simulink model "TVModel_Simulation_21"  (R2021b)
settings: Solver=FixedStepDiscrete  StartTime=0.0  StopTime=250  FixedStep=0.02  MaxStep=0.01  RelTol=1e-3
undefined symbols (not defined in the file or in its folder): MB, TV, TV_OLD
libraries: simulink x22, simulink_extras x14, eeGeneralControl x13, slpidlib x8, fuzblock x4, controlLib x4, cstblocks x3, dspstat3 x2, eeSlidingModeController x1, sharedTrackingLibrary x1
(part 5 of 9)

== system TVModel_Simulation_21/Subsystem/Subsystem1/Torque Distribution/MPC/ PRE LUDO/Mz = 0 Bound logic ==
  In Bus Element13 : Inport  PortName=brake_signal  Element=regen
  YRD : Inport  Port=2
  In Bus Element1 : Inport  Port=3  PortName=driver_inputs  Element=throttle
  " " : Constant  Value=0.95
  "  " : Constant  Value=TV.LV.GENERAL.ThrottleThresh
  "             " : Constant  Value=TV.LV.GENERAL.YRDTresh
  AND : Logic  IconShape=distinctive  AllPortsSameDT=off  OutDataTypeStr=boolean
  AND1 : Logic  IconShape=distinctive  AllPortsSameDT=off  OutDataTypeStr=boolean
  AND2 : Logic  IconShape=distinctive  AllPortsSameDT=off  OutDataTypeStr=boolean
  Abs : Abs
  Constant : Constant  Value=TV.LV.GENERAL.BrakeThresh
  Constant1 : Constant  Value=10
  Data Type Conversion : DataTypeConversion  OutDataTypeStr=double
  Data Type Conversion1 : DataTypeConversion  OutDataTypeStr=double
  Discrete FIR Filter : DiscreteFir  Coefficients=ones(1,TV.MPC.N/TV.MPC.T*0.2)
  Gain : Gain  Gain=2
  Less Than : RelationalOperator  Operator=<=  OutDataTypeStr=fixdt(1,16)  RndMeth=Simplest
  Less Than1 : RelationalOperator  OutDataTypeStr=boolean  RndMeth=Simplest
  Less Than2 : RelationalOperator  Operator=<  OutDataTypeStr=boolean  RndMeth=Simplest
  Less Than3 : RelationalOperator  Operator=<  OutDataTypeStr=boolean  RndMeth=Simplest
  Less Than4 : RelationalOperator  OutDataTypeStr=boolean  RndMeth=Simplest
  Sum : Sum
  flag : Outport
  wires:
  Less Than/1 -> Discrete FIR Filter/1
  Constant1/1 -> Less Than4/2
  Less Than4/1 -> AND/1, AND1/2
  Discrete FIR Filter/1 -> Less Than4/1
  "  "/1 -> Less Than1/2
  "             "/1 -> Less Than/2
  Abs/1 -> Less Than/1
  YRD/1 -> Abs/1
  In Bus Element1/1 -> Less Than1/1
  Less Than1/1 -> AND/2
  In Bus Element13/1 -> Less Than3/2, Less Than2/1
  " "/1 -> Less Than2/2
  AND1/1 -> Data Type Conversion1/1
  Gain/1 -> Sum/1
  AND/1 -> Data Type Conversion/1
  Sum/1 -> flag/1
  Data Type Conversion/1 -> Sum/2
  Data Type Conversion1/1 -> Gain/1
  AND2/1 -> AND1/1
  Less Than2/1 -> AND2/1
  Less Than3/1 -> AND2/2
  Constant/1 -> Less Than3/1

== system TVModel_Simulation_21/Subsystem/Subsystem1/Torque Distribution/MPC/ PRE LUDO/Power Calculation Post ==
  Motor_Torque : Inport  OutDataTypeStr=double  PortDimensions=4
  In Bus Element34 : Inport  Port=2  PortName=dynamics_data  Element=omega_wheels
  In Bus Element2 : Inport  Port=2  PortName=dynamics_data  Element=omega_wheels
  "     " : Gain  Gain=TV.LV.inv_efficiency
  "      " : Gain  Gain=1/TV.LV.inv_efficiency
  Divide : Product  Inputs=*/*
  Gain2 : Gain  Gain=TV.CAR.Tau
  Power to engines : Subsystem
  Saturation : Saturate  UpperLimit=19900*pi/30  LowerLimit=100*pi/30
  Sum of Elements : Sum  Inputs=+
  Switch3 : Switch  Criteria=u2 > Threshold
  Terminator : Terminator
  wires:
  Divide/1 -> Sum of Elements/1
  Saturation/1 -> Divide/1, Power to engines/1(omega_motor)
  Power to engines/1(Efficiency) -> "      "/1, "     "/1
  "      "/1 -> Switch3/3  "Braking"
  "     "/1 -> Switch3/1  "Driving"
  Motor_Torque/1 -> Power to engines/2(Torque), Divide/3
  In Bus Element34/1 -> Gain2/1
  Gain2/1 -> Saturation/1
  In Bus Element2/1 -> Switch3/2
  Switch3/1 -> Divide/2
  Sum of Elements/1 -> Terminator/1  "p_el_post"

== system TVModel_Simulation_21/Subsystem/Subsystem1/Torque Distribution/MPC/ PRE LUDO/Power Calculation Pre ==
  Motor_Torque : Inport  OutDataTypeStr=double  PortDimensions=4
  In Bus Element34 : Inport  Port=2  PortName=dynamics_data  Element=omega_wheels
  In Bus Element2 : Inport  Port=2  PortName=dynamics_data  Element=omega_wheels
  "     " : Gain  Gain=TV.LV.inv_efficiency
  "      " : Gain  Gain=1/TV.LV.inv_efficiency
  Divide : Product  Inputs=*/*
  Gain2 : Gain  Gain=TV.CAR.Tau
  Power to engines : Subsystem
  Saturation : Saturate  UpperLimit=19900*pi/30  LowerLimit=100*pi/30
  Sum of Elements : Sum  Inputs=+
  Switch3 : Switch  Criteria=u2 > Threshold
  Terminator : Terminator
  wires:
  Power to engines/1(Efficiency) -> "      "/1, "     "/1
  "      "/1 -> Switch3/3  "Braking"
  "     "/1 -> Switch3/1  "Driving"
  Motor_Torque/1 -> Divide/3, Power to engines/2(Torque)
  In Bus Element34/1 -> Gain2/1
  Gain2/1 -> Saturation/1
  In Bus Element2/1 -> Switch3/2
  Sum of Elements/1 -> Terminator/1  "p_el_pre"
  Saturation/1 -> Divide/1, Power to engines/1(omega_motor)
  Switch3/1 -> Divide/2
  Divide/1 -> Sum of Elements/1

== system TVModel_Simulation_21/Subsystem/Subsystem1/Torque Distribution/MPC/ PRE LUDO/Steer_activation ==
  front_wheel_angle : Inport
  Constant : Constant  Value=TV.SIGNALS.SETTINGS.MzLimit
  Product : Product
  Steer Activation : Subsystem
  Mz_Lim : Outport
  wires:
  Constant/1 -> Product/2
  Steer Activation/1(epsilon) -> Product/1  "epsilon"
  Product/1 -> Mz_Lim/1  "Mz_Lim"
  front_wheel_angle/1 -> Steer Activation/1(front_wheel_angle)

== system TVModel_Simulation_21/Subsystem/Subsystem1/Torque Distribution/MPC/ Parameter Bus /Bus p ==
  In : Inport
  C Function : CFunction  OutputCode=|
      | int i,j;
      | for (i = 0; i < N; i++) {
      |  for (j = 0; j < np; j++) {
      |   out_x[i*np+j] = in_x[j];
      |  }
      | }
  Constant1 : Constant  Value=TV.MPC.N + 1  OutDataTypeStr=uint8  SampleTime=TV.MPC.T/TV.MPC.N
  Constant3 : Constant  Value=TV.MPC.np  OutDataTypeStr=uint8  SampleTime=TV.MPC.T/TV.MPC.N
  Rate Transition3 : RateTransition  OutPortSampleTime=TV.MPC.T/TV.MPC.N
  TV_Info : Outport
  wires:
  Constant1/1 -> C Function/2
  C Function/1 -> TV_Info/1
  Constant3/1 -> C Function/3
  Rate Transition3/1 -> C Function/1
  In/1 -> Rate Transition3/1

== system TVModel_Simulation_21/Subsystem/Subsystem1/Torque Distribution/MPC/Faults Detection/MPC ==
  X1 : Inport
  Action Port : ActionPort  ActionPortLabel=if(u1 == 1)
  Out1 : Outport
  wires:
  X1/1 -> Out1/1

== system TVModel_Simulation_21/Subsystem/Subsystem1/Torque Distribution/MPC/Faults Detection/Simple torque ==
  In Bus Element11 : Inport  PortName=driver_inputs
  In Bus Element10 : Inport  Port=2  PortName=dynamics_data
  In Bus Element13 : Inport  Port=3  PortName=brake_signal
  In Bus Element12 : Inport  Port=4  PortName=hv
  In Bus torque_map1 : Inport  Port=5  PortName=car_settings
  Bus Element In : Inport  Port=6  PortName=Tire_Bounds
  Action Port : ActionPort  ActionPortLabel=elseif(u1 == 2)
  No_TV : Subsystem
  Out1 : Outport
  wires:
  Bus Element In/1 -> No_TV/6(Tire_Bounds)
  No_TV/1(Output) -> Out1/1
  In Bus Element11/1 -> No_TV/4(driver_inputs)
  In Bus Element10/1 -> No_TV/1(dynamics_data)
  In Bus Element12/1 -> No_TV/3(hv)
  In Bus Element13/1 -> No_TV/2(brake_signal)
  In Bus torque_map1/1 -> No_TV/5(car_settings)

== system TVModel_Simulation_21/Subsystem/Subsystem1/Torque Distribution/MPC/Faults Detection/Subsystem ==
  OCP Status : Inport
  In Bus Element2 : Inport  Port=2  PortName=dynamics_data  Element=vx
  Backup Map : Subsystem  TreatAsAtomicUnit=on
  Constant : Constant  Value=2
  Constant1 : Constant  Value=TV.MPC.N/TV.MPC.T*0.1-1
  Constant2 : Constant  Value=4
  Data Type Conversion : DataTypeConversion  OutDataTypeStr=uint8  RndMeth=Nearest
  Discrete FIR Filter : DiscreteFir  Coefficients=ones(1,TV.MPC.N/TV.MPC.T*0.1)
  Equal : RelationalOperator  Operator===  OutDataTypeStr=boolean  RndMeth=Simplest
  If : If  IfExpression=u1 == 0
  Less Than1 : RelationalOperator  OutDataTypeStr=boolean  RndMeth=Simplest
  Merge : Merge
  Selected Map : Subsystem  TreatAsAtomicUnit=on
  Switch : Switch  Criteria=u2 > Threshold  Threshold=TV.LV.GENERAL.VxTresh
  TV Mode Selection : Outport
  wires:
  Data Type Conversion/1 -> Discrete FIR Filter/1
  Constant2/1 -> Equal/2
  OCP Status/1 -> Equal/1
  Equal/1 -> Data Type Conversion/1
  Constant/1 -> Switch/3
  Switch/1 -> TV Mode Selection/1
  In Bus Element2/1 -> Switch/2
  Merge/1 -> Switch/1
  Discrete FIR Filter/1 -> Less Than1/1
  Constant1/1 -> Less Than1/2
  Less Than1/1 -> If/1
  If/1 -> Selected Map/Action
  Selected Map/1(Out1) -> Merge/1
  If/2 -> Backup Map/Action
  Backup Map/1(Out1) -> Merge/2

== system TVModel_Simulation_21/Subsystem/Subsystem1/Torque Distribution/MPC/Mz Generation/Steer Activation ==
  front_wheel_angle : Inport
  In Bus Element2 : Inport  Port=2  PortName=dynamics_data  Element=vx
  AND : Logic  Commented=on  IconShape=distinctive  AllPortsSameDT=off  OutDataTypeStr=boolean
  AND1 : Logic  Commented=on  IconShape=distinctive  AllPortsSameDT=off  OutDataTypeStr=boolean
  Abs : Abs
  Constant : Constant  Commented=on  Value=TV.LV.GENERAL.VxTresh
  Constant1 : Constant  Value=2*pi/180
  Constant4 : Constant  Value=pi/180/2
  Delay : Delay  Commented=on  DelayLength=5
  First Activation : Subsystem  Commented=on
  If : If  Commented=on  IfExpression=u1 == 1
  If Action Subsystem : Subsystem  Commented=on  TreatAsAtomicUnit=on
  If Action Subsystem1 : Subsystem  Commented=on  TreatAsAtomicUnit=on
  Less Than : RelationalOperator  Operator=<=  OutDataTypeStr=boolean  RndMeth=Simplest
  Less Than1 : RelationalOperator  Commented=on  OutDataTypeStr=boolean  RndMeth=Simplest
  Less Than2 : RelationalOperator  Operator=<  OutDataTypeStr=boolean  RndMeth=Simplest
  Merge : Merge  Commented=on
  S-R Flip-Flop : simulink_extras/Flip Flops/S-R Flip-Flop  initial_condition=0
  Terminator : Terminator
  epsilon : Outport
  wires:
  If/1 -> If Action Subsystem1/Action
  If Action Subsystem/1(Epsilon) -> Merge/2
  If Action Subsystem1/1(epsilon) -> Merge/1
  First Activation/1(OUt) -> If/1  "u1"
  S-R Flip-Flop/1 -> First Activation/1(In), epsilon/1, If Action Subsystem1/1(Inport), Delay/1, If Action Subsystem/1(Inport)  "Q"
  If/2 -> If Action Subsystem/Action
  front_wheel_angle/1 -> Abs/1
  Constant1/1 -> Less Than/1
  S-R Flip-Flop/2 -> Terminator/1
  Less Than2/1 -> S-R Flip-Flop/2, AND/1  "reset"
  Less Than/1 -> S-R Flip-Flop/1  "set"
  Delay/1 -> AND/2
  Abs/1 -> Less Than/2, Less Than2/1
  Constant4/1 -> Less Than2/2
  Merge/1 -> AND1/1  "epsilon"
  Less Than1/1 -> AND1/2
  Constant/1 -> Less Than1/2
  In Bus Element2/1 -> Less Than1/1

== system TVModel_Simulation_21/Subsystem/Subsystem1/Torque Distribution/MPC/Polytopic Constraints/Driver Inputs ==
  In Bus Element35 : Inport  PortName=brake_signal  Element=regen
  In Bus Element2 : Inport  Port=2  PortName=driver_inputs  Element=throttle
  In Bus torque_map : Inport  Port=3  PortName=Car_Settings  Element=torque_map
  Bus Element In1 : Inport  Port=4  PortName=ubx  Element=ubx
  Bus Element In2 : Inport  Port=4  PortName=ubx  Element=lbx
  " " : Logic  Operator=XOR  IconShape=distinctive  AllPortsSameDT=off  OutDataTypeStr=boolean
  "Accelerator Mapping " : Subsystem
      settings: PortSchema="{\"entries\":[{\"content\":{\"sides\":[{\"content\":{\"connectorIds\":[\"In1\"]},\"type\":\"ConnectorPlacement.EquallySpacedRectSide\",\"uuid\":\"12eec289-8173-4d00-9637-a8f11e8894d3\"},{\"content\":{\"connectorIds\":[\"Out1\"],\"side\":\"RIGHT\"},\"type\":\"ConnectorPlacement.EquallySpacedRectSide\",\"uuid\":\"db75e905-0694-4773-89a3-439123e45b7e\"},{\"content\":{\"connectorIds\":[\"Out2\"],\"side\":\"TOP\"},\"type\":\"ConnectorPlacement.EquallySpacedRectSide\",\"uuid\":\"1c38e3d9-f7d7-40f1-94e6-0479f4c62d9d\"}]},\"type\":\"ConnectorPlacement.EquallySpacedConnector\",\"uuid\":\"6d4996fb-8621-4156-91e1-8a66b5180382\"}],\"packageUris\":[\"http://schema.mathworks.com/mf0/Connector/R2020b\"],\"version\":\"1.0\"}"
  Constant1 : Constant  Value=TV.LV.GENERAL.BrakeThresh
  Constant10 : Constant  Value=TV.LV.TORQUE.T_nominal_motor
  Constant2 : Constant  Value=TV.LV.GENERAL.ThrottleThresh
  Constant9 : Constant  Value=TV.LV.TORQUE.T_peak_motor
  Gain1 : Gain  Gain=4
  Gain2 : Gain  Gain=0.99
  Gain3 : Gain
  Less Than : RelationalOperator  OutDataTypeStr=boolean  RndMeth=Simplest
  Less Than1 : RelationalOperator  OutDataTypeStr=boolean  RndMeth=Simplest
  MATLAB Function3 : MATLAB Function  TreatAsAtomicUnit=on
  MATLAB Function4 : MATLAB Function  TreatAsAtomicUnit=on
  Multiport Switch1 : MultiPortSwitch  DataPortOrder=Specify indices  Inputs={TV.LV.TORQUE.T_peak_setting,TV.LV.TORQUE.T_nominal_setting}  DataPortIndices={TV.LV.TORQUE.T_peak_setting,TV.LV.TORQUE.T_nominal_setting}
  Product : Product
  Product1 : Product
  Saturation Dynamic : simulink/Discontinuities/Saturation Dynamic  OutMin=[]  OutMax=[]  OutDataTypeStr=Inherit: Same as second input  OutDataType=fixdt(1, 16)  OutScaling=2^-10  DoSatur=off
  Subtract1 : Sum  Inputs=+-
  Out Bus Element : Outport  PortName=percentage  Element=95
  Out Bus Element1 : Outport  PortName=percentage  Element=105
  Out Bus Element2 : Outport  Port=2  PortName=TV_Info  Element=Accelerator_Mapping
  wires:
  Product1/1 -> Product/1
  " "/1 -> Product1/1
  Constant9/1 -> Multiport Switch1/2
  Product/1 -> Saturation Dynamic/2  "g_requested"
  Subtract1/1 -> Product1/2
  Multiport Switch1/1 -> Gain1/1
  Constant10/1 -> Multiport Switch1/3
  Constant2/1 -> Less Than1/2
  "Accelerator Mapping "/1(mapped_acc) -> Subtract1/1
  In Bus torque_map/1 -> Multiport Switch1/1
  In Bus Element35/1 -> Less Than/1, Subtract1/2  "regen"
  Less Than1/1 -> " "/2
  Constant1/1 -> Less Than/2
  In Bus Element2/1 -> "Accelerator Mapping "/1(acc), Less Than1/1
  Less Than/1 -> " "/1
  Gain1/1 -> Product/2
  "Accelerator Mapping "/2(TV_Info) -> Out Bus Element2/1
  Gain3/1 -> Out Bus Element1/1
  MATLAB Function4/1(ug_saturation) -> Saturation Dynamic/1
  Bus Element In2/1 -> MATLAB Function3/1(lbx)
  MATLAB Function3/1(lg_saturation) -> Saturation Dynamic/3
  Saturation Dynamic/1 -> Gain3/1, Gain2/1  "yg"
  Gain2/1 -> Out Bus Element/1
  Bus Element In1/1 -> MATLAB Function4/1(ubx)

== system TVModel_Simulation_21/Subsystem/Subsystem1/Torque Distribution/MPC/Polytopic Constraints/Driver g ==
  In Bus Element1 : Inport  PortName=brake_signal
  In Bus Element : Inport  Port=2  PortName=percentage  Element=95
  In Bus Element2 : Inport  Port=2  PortName=percentage  Element=95
  In Bus Element4 : Inport  Port=2  PortName=percentage  Element=105
  In Bus Element5 : Inport  Port=2  PortName=percentage  Element=105
  In Bus Element3 : Inport  Port=3  PortName=driver_inputs
  Coasting : Subsystem
      settings: PortSchema="{\"entries\":[{\"content\":{\"sides\":[{\"content\":{\"connectorIds\":[\"In1\",\"In2\"]},\"type\":\"ConnectorPlacement.EquallySpacedRectSide\",\"uuid\":\"12822615-03ad-45f6-8c43-45acae00b3c9\"},{\"content\":{\"connectorIds\":[\"Out1\"],\"side\":\"RIGHT\"},\"type\":\"ConnectorPlacement.EquallySpacedRectSide\",\"uuid\":\"651d1d31-9a4c-422b-aacb-e7edf3ade298\"},{\"content\":{\"connectorIds\":[\"Out2\"],\"side\":\"TOP\"},\"type\":\"ConnectorPlacement.EquallySpacedRectSide\",\"uuid\":\"d0f71465-89ce-4a1f-947c-d935b63c1581\"}]},\"type\":\"ConnectorPlacement.EquallySpacedConnector\",\"uuid\":\"d07c68d3-c928-4ca4-a746-c386ba32e252\"}],\"packageUris\":[\"http://schema.mathworks.com/mf0/Connector/R2020b\"],\"version\":\"1.0\"}"
  Engine Brake : Constant  Value=-TV.SIGNALS.SETTINGS.EngineBrake*TV.LV.TORQUE.T_nominal_motor*4
  Max : MinMax  Function=max  Inputs=2
  Max1 : MinMax  Inputs=2
  Switch2 : Switch  Criteria=u2 > Threshold
  ug_driver : Outport
  lg_driver : Outport  Port=2
  Out Bus Element1 : Outport  Port=3  PortName=TV_Info  Element=Coasting
  wires:
  In Bus Element3/1 -> Coasting/1(driver_inputs)
  In Bus Element1/1 -> Coasting/2(brake_signal)
  Switch2/1 -> lg_driver/1
  In Bus Element/1 -> Max1/1
  Max1/1 -> Switch2/3
  Engine Brake/1 -> Switch2/1
  Coasting/1(coasting_flag) -> Switch2/2
  In Bus Element2/1 -> Max/1
  In Bus Element4/1 -> Max1/2
  In Bus Element5/1 -> Max/2
  Coasting/2(TV_Info) -> Out Bus Element1/1
  Max/1 -> ug_driver/1

== system TVModel_Simulation_21/Subsystem/Subsystem1/Torque Distribution/MPC/Polytopic Constraints/Power Limits Negative ==
  In Bus Element5 : Inport  PortName=hv  Element=cooling.battery.Power_limits [W]
  Gain : Gain  Gain=1/1000
  IC : InitialCondition  Value=-35000
  Max Regen : Saturate  UpperLimit=40000  LowerLimit=0
  Selector : Selector  InputPortWidth=2  IndexOptions=Index vector (dialog)  Indices=[1]  OutputSizes=1
  Unary Minus1 : UnaryMinus
  lg_power : Outport
  wires:
  Unary Minus1/1 -> IC/1  "lPowerLimit"
  Max Regen/1 -> Unary Minus1/1
  In Bus Element5/1 -> Selector/1
  Selector/1 -> Max Regen/1
  IC/1 -> Gain/1
  Gain/1 -> lg_power/1

== system TVModel_Simulation_21/Subsystem/Subsystem1/Torque Distribution/MPC/Polytopic Constraints/Power Limits Positive ==
  In Bus Element5 : Inport  PortName=hv  Element=cooling.battery.Power_limits [W]
  Gain : Gain  Gain=1/1000
  IC1 : InitialCondition  Value=80000
  Selector1 : Selector  InputPortWidth=2  IndexOptions=Index vector (dialog)  Indices=[2]  OutputSizes=1
  ug_power : Outport
  wires:
  In Bus Element5/1 -> Selector1/1
  Selector1/1 -> IC1/1  "uPowerLimit"
  IC1/1 -> Gain/1
  Gain/1 -> ug_power/1

== system TVModel_Simulation_21/Subsystem/Subsystem1/Torque Distribution/MPC/Polytopic Constraints/Subsystem ==
  Torque : Inport
  Abs1 : Abs
  Abs3 : Abs
  Selector : Selector  InputPortWidth=4  IndexOptions=Index vector (dialog)  Indices=[2]  OutputSizes=1
  Selector1 : Selector  InputPortWidth=4  IndexOptions=Index vector (dialog)  Indices=[1]  OutputSizes=1
  Torque1 : InportShadow
  Right : Outport
  Left : Outport  Port=2
  wires:
  Torque1/1 -> Selector1/1
  Selector1/1 -> Abs3/1
  Selector/1 -> Abs1/1
  Torque/1 -> Selector/1
  Abs1/1 -> Right/1
  Abs3/1 -> Left/1

== system TVModel_Simulation_21/Subsystem/Subsystem1/Torque Distribution/MPC/Polytopic Constraints/Subsystem1 ==
  Torque : Inport
  Abs1 : Abs
  Abs3 : Abs
  Selector : Selector  InputPortWidth=4  IndexOptions=Index vector (dialog)  Indices=[2]  OutputSizes=1
  Selector1 : Selector  InputPortWidth=4  IndexOptions=Index vector (dialog)  Indices=[1]  OutputSizes=1
  Torque1 : InportShadow
  Unary Minus : UnaryMinus
  Unary Minus1 : UnaryMinus
  Right : Outport
  Left : Outport  Port=2
  wires:
  Abs1/1 -> Unary Minus/1
  Torque/1 -> Selector/1
  Selector/1 -> Abs1/1
  Selector1/1 -> Abs3/1
  Torque1/1 -> Selector1/1
  Abs3/1 -> Unary Minus1/1
  Unary Minus/1 -> Right/1
  Unary Minus1/1 -> Left/1

== system TVModel_Simulation_21/Subsystem/Subsystem1/Torque Distribution/MPC/States Constraints/Anti reverse wheelspin ==
  lbx_in : Inport  PortDimensions=4
  In Bus Element4 : Inport  Port=2  PortName=slip_ratio
  In Bus Element1 : Inport  Port=2  PortName=slip_ratio
  Constant : Constant  Value=-0.6
  Constant1 : Constant  Value=-0.3
  Less Than : RelationalOperator  Operator=<=  OutDataTypeStr=boolean  RndMeth=Simplest
  Less Than1 : RelationalOperator  OutDataTypeStr=boolean  RndMeth=Simplest
  NOT : Logic  Operator=NOT  IconShape=distinctive  AllPortsSameDT=off  OutDataTypeStr=boolean
  Product : Product
  S-R Flip Flops : Subsystem
  Terminator : Terminator
  lbx_out : Outport  PortDimensions=4
  wires:
  NOT/1 -> Terminator/1  "AntiWheelSpin_Activation_Flag"
  S-R Flip Flops/1(Out1) -> Product/2, NOT/1
  Less Than1/1 -> S-R Flip Flops/2(Reset)
  Less Than/1 -> S-R Flip Flops/1(Set)
  Constant1/1 -> Less Than1/2
  In Bus Element1/1 -> Less Than1/1
  Product/1 -> lbx_out/1
  lbx_in/1 -> Product/1
  In Bus Element4/1 -> Less Than/1
  Constant/1 -> Less Than/2

== system TVModel_Simulation_21/Subsystem/Subsystem1/Torque Distribution/MPC/States Constraints/Brake & ESP ==
  ubx_in : Inport
  In Bus Element13 : Inport  Port=2  PortName=brake_signal  Element=regen
  Constant : Constant
  Constant1 : Constant  Value=0
  Product : Product
  Switch : Switch  Criteria=u2 > Threshold  Threshold=0.95
  ubx_out : Outport
  wires:
  Product/1 -> ubx_out/1
  Switch/1 -> Product/2
  ubx_in/1 -> Product/1
  Constant1/1 -> Switch/1
  Constant/1 -> Switch/3
  In Bus Element13/1 -> Switch/2

== system TVModel_Simulation_21/Subsystem/Subsystem1/Torque Distribution/MPC/States Constraints/Low YRD ==
  ubx_in : Inport
  lbx_max : Inport  Port=2
  lbx_in : Inport  Port=3
  Demux : Demux
  Demux1 : Demux
  Mux : Mux  Inputs=9
  bounds : Outport
  wires:
  lbx_max/1 -> Mux/5
  Demux/4 -> Mux/4
  Demux/3 -> Mux/3
  Demux/2 -> Mux/2
  Demux/1 -> Mux/1
  ubx_in/1 -> Demux/1
  Mux/1 -> bounds/1
  Demux1/3 -> Mux/8
  lbx_in/1 -> Demux1/1
  Demux1/2 -> Mux/7
  Demux1/4 -> Mux/9
  Demux1/1 -> Mux/6

== system TVModel_Simulation_21/Subsystem/Subsystem1/Torque Distribution/MPC/States Constraints/Tire Bounds ==
  In Bus Element : Inport  PortName=fz
  In Bus Element2 : Inport  PortName=fz
  In Bus Element1 : Inport  Port=2  PortName=slip_angle
  In Bus Element3 : Inport  Port=2  PortName=slip_angle
  In Bus Element4 : Inport  Port=3  PortName=dynamics_data
  2-D Lookup Table : Lookup_n-D  BreakpointsForDimension1=TV.LUT.MPC_Lut.control_bound_dry.Fz  BreakpointsForDimension2=TV.LUT.MPC_Lut.control_bound_dry.alpha  Table=TV.LUT.MPC_Lut.control_bound_dry.Fx_target_positive  InternalRulePriority=Speed  RndMeth=Simplest  InputSameDT=on
      settings: InputPortMap=u0,u1
  2-D Lookup Table1 : Lookup_n-D  BreakpointsForDimension1=TV.LUT.MPC_Lut.control_bound_dry.Fz  BreakpointsForDimension2=TV.LUT.MPC_Lut.control_bound_dry.alpha  Table=TV.LUT.MPC_Lut.control_bound_dry.Fx_target_negative  InternalRulePriority=Speed  RndMeth=Simplest  InputSameDT=on
      settings: InputPortMap=u0,u1
  Gain : Gain  Gain=TV.CAR.rs/TV.CAR.Tau
  Gain1 : Gain  Gain=TV.CAR.rs/TV.CAR.Tau
  Hydraulic brakes : Subsystem
  LMUx Correction : Subsystem
      settings: PortSchema="{\"entries\":[{\"content\":{\"sides\":[{\"content\":{\"connectorIds\":[]},\"type\":\"ConnectorPlacement.EquallySpacedRectSide\",\"uuid\":\"3584feb2-5a88-411e-904a-cebd49175db1\"},{\"content\":{\"connectorIds\":[\"Out1\"],\"side\":\"RIGHT\"},\"type\":\"ConnectorPlacement.EquallySpacedRectSide\",\"uuid\":\"3ab4f304-c705-48db-a675-7c67b0246c6a\"},{\"content\":{\"connectorIds\":[\"Out2\"],\"side\":\"TOP\"},\"type\":\"ConnectorPlacement.EquallySpacedRectSide\",\"uuid\":\"35f1ab2e-6666-4377-9bcf-c0062baa00ab\"}]},\"type\":\"ConnectorPlacement.EquallySpacedConnector\",\"uuid\":\"03f15aa2-f62f-4666-8bb4-1f7a61fcffbb\"}],\"packageUris\":[\"http://schema.mathworks.com/mf0/Connector/R2020b\"],\"version\":\"1.0\"}"
  Product : Product
  Product1 : Product
  Saturation : Saturate  UpperLimit=0  LowerLimit=-inf
  Saturation1 : Saturate  UpperLimit=+inf  LowerLimit=0
  tire_ubx : Outport
  tire_lbx : Outport  Port=2
  Out Bus Element1 : Outport  Port=3  PortName=TV_Info  Element=tire_lbx
  Out Bus Element2 : Outport  Port=3  PortName=TV_Info  Element=tire_ubx
  Out Bus Element3 : Outport  Port=3  PortName=TV_Info  Element=LMUx_Correction
  wires:
  In Bus Element/1 -> 2-D Lookup Table/1
  In Bus Element1/1 -> 2-D Lookup Table/2
  In Bus Element2/1 -> 2-D Lookup Table1/1
  In Bus Element3/1 -> 2-D Lookup Table1/2
  Saturation1/1 -> tire_ubx/1, Out Bus Element2/1
  2-D Lookup Table1/1 -> Gain1/1
  In Bus Element4/1 -> Hydraulic brakes/2(dynamics_data)
  Gain1/1 -> Product1/2
  Product/1 -> Saturation1/1
  Gain/1 -> Product/1
  Hydraulic brakes/1(tire_lbx_out) -> Saturation/1
  Product1/1 -> Hydraulic brakes/1(tire_lbx_in)
  LMUx Correction/1(lmux) -> Product/2, Product1/1
  2-D Lookup Table/1 -> Gain/1
  Saturation/1 -> tire_lbx/1, Out Bus Element1/1
  LMUx Correction/2(TV_Info) -> Out Bus Element3/1

== system TVModel_Simulation_21/Subsystem/Subsystem1/Torque Distribution/MPC/USEFUL STUFFFF/Extended Kalman Filter ==
  Motor_Torque : Inport
  In Bus Element4 : Inport  Port=2  PortName=slip_ratio
  In Bus Element : Inport  Port=3  PortName=dynamics_data  Element=vx
  In Bus Element1 : Inport  Port=3  PortName=dynamics_data  Element=vy
  In Bus Element2 : Inport  Port=3  PortName=dynamics_data  Element=yaw_rate
  In Bus Element11 : Inport  Port=4  PortName=front_wheel_angles
  " Parameter Bus " : Subsystem
  Band-Limited White Noise : simulink/Sources/Band-Limited White Noise  Cov=0.00005  Ts=0.01  seed=[23341]
  Band-Limited White Noise1 : simulink/Sources/Band-Limited White Noise  Cov=0.000001  Ts=0.01  seed=[23341]
  Band-Limited White Noise2 : simulink/Sources/Band-Limited White Noise  Cov=0.00001  Ts=0.01  seed=[85]
  Extended Kalman Filter : sharedTrackingLibrary/Extended Kalman Filter  StateTransitionFcn=state_update_kalman  HasStateTransitionJacobianFcn=off  HasAdditiveProcessNoise=Additive  ProcessNoise=diag(0.1*[0.1,0.1,0.1])  HasTimeVaryingProcessNoise=off  HasStateTransitionFcnExtraArgument=1  InitialState=[0,0,0];  InitialStateCovariance=diag(0.1*[0.1,0.1,0.1])  MeasurementFcn1=measurement_kalman  HasMeasurementJacobianFcn1=off  HasMeasurementEnablePort1=off  HasAdditiveMeasurementNoise1=Additive  MeasurementNoise1=diag(0.1*[0.01,0.01,1])  HasTimeVaryingMeasurementNoise1=off  HasMeasurementFcnExtraArgument1=0  HasMeasurementWrapping1=off  MeasurementFcn2=myMeasurementFcn  HasMeasurementJacobianFcn2=off  HasMeasurementEnablePort2=off  HasAdditiveMeasurementNoise2=Additive  MeasurementNoise2=1  HasTimeVaryingMeasurementNoise2=off  HasMeasurementFcnExtraArgument2=0  HasMeasurementWrapping2=off  MeasurementFcn3=myMeasurementFcn  HasMeasurementJacobianFcn3=off  HasMeasurementEnablePort3=off  HasAdditiveMeasurementNoise3=Additive  MeasurementNoise3=1  HasTimeVaryingMeasurementNoise3=off  HasMeasurementFcnExtraArgument3=0  HasMeasurementWrapping3=off  MeasurementFcn4=myMeasurementFcn  HasMeasurementJacobianFcn4=off  HasMeasurementEnablePort4=off  HasAdditiveMeasurementNoise4=Additive  MeasurementNoise4=1  HasTimeVaryingMeasurementNoise4=off  HasMeasurementFcnExtraArgument4=0  HasMeasurementWrapping4=off  MeasurementFcn5=myMeasurementFcn  HasMeasurementJacobianFcn5=off  HasMeasurementEnablePort5=off  HasAdditiveMeasurementNoise5=Additive  MeasurementNoise5=1  HasTimeVaryingMeasurementNoise5=off  HasMeasurementFcnExtraArgument5=0  HasMeasurementWrapping5=off  EnableMultirate=off  StateTransitionFcnSampleTime=1  MeasurementFcn1SampleTime=1  MeasurementFcn2SampleTime=1  MeasurementFcn3SampleTime=1  MeasurementFcn4SampleTime=1  MeasurementFcn5SampleTime=1  UseCurrentEstimator=on  OutputStateCovariance=off  DataType=double  SampleTime=TV.MPC.T/TV.MPC.N  NumberOfMeasurements=1
      settings: SourceProductBaseCode=AE,PW,CT,DR,TF,ID,LP,NV,AR,RO,RR,UV,VE
  Mux : Mux  Inputs=3
  Rate Transition{,1..3} (4 alike) : RateTransition  OutPortSampleTime=TV.MPC.T/TV.MPC.N
  Sum : Sum  Inputs=++|
  Sum1 : Sum  Inputs=++|
  Sum2 : Sum  Inputs=++|
  measurement_kalman_simulink : Subsystem  Commented=on  TreatAsAtomicUnit=on
  state_update_kalman_simulink : Subsystem  Commented=on  TreatAsAtomicUnit=on
  vx_meas : Outport
  vy_meas : Outport  Port=2
  yaw_rate_meas : Outport  Port=3
  xhat : Outport  Port=4
  Out Bus Element1 : Outport  Port=5  PortName=TV_Info  Element=xhat_ext
  wires:
  In Bus Element11/1 -> " Parameter Bus "/3(front_wheel_angles)
  Motor_Torque/1 -> " Parameter Bus "/1(Motor_Torque)
  In Bus Element4/1 -> " Parameter Bus "/2(slip_ratio)
  Rate Transition3/1 -> yaw_rate_meas/1, Mux/3
  Sum2/1 -> Rate Transition3/1  "r_meas"
  Rate Transition2/1 -> vy_meas/1, Mux/2
  Sum1/1 -> Rate Transition2/1  "vy_meas"
  Sum/1 -> Rate Transition1/1  "vx_meas"
  Rate Transition1/1 -> Mux/1, vx_meas/1
  Band-Limited White Noise/1 -> Sum2/1
  In Bus Element2/1 -> Sum2/2
  Band-Limited White Noise1/1 -> Sum1/1
  In Bus Element1/1 -> Sum1/2
  Band-Limited White Noise2/1 -> Sum/1
  In Bus Element/1 -> Sum/2
  Extended Kalman Filter/1 -> Out Bus Element1/1, xhat/1
  Mux/1 -> Extended Kalman Filter/2
  " Parameter Bus "/1(p) -> Rate Transition/1
  Rate Transition/1 -> Extended Kalman Filter/1, state_update_kalman_simulink/1(Parameters)

== system TVModel_Simulation_21/Subsystem/Subsystem1/Torque Distribution/MPC/USEFUL STUFFFF/Power Limiter ==
  In Bus Element5 : Inport  PortName=hv
  In Bus Element4 : Inport  PortName=hv
  In Bus Element3 : Inport  PortName=hv  Element=Pmax_tractive
  In Bus Element1 : Inport  PortName=hv  Element=current
  In Bus Element2 : Inport  PortName=hv  Element=voltage
  If : If  IfExpression=u1 < 0
  If Action Subsystem : Subsystem  TreatAsAtomicUnit=on
  If Action Subsystem1 : Subsystem  TreatAsAtomicUnit=on
  Merge : Merge
  Product : Product
  Subtract : Sum  Inputs=+-
  Out1 : Outport
  wires:
  In Bus Element1/1 -> Product/1  "hv"
  In Bus Element2/1 -> Product/2  "hv"
  In Bus Element3/1 -> Subtract/1  "hv"
  Product/1 -> Subtract/2
  Subtract/1 -> If Action Subsystem/2(Inport), If/1
  If/1 -> If Action Subsystem/Action
  If/2 -> If Action Subsystem1/Action
  If Action Subsystem1/1(Out1) -> Merge/2
  If Action Subsystem/1(Out1) -> Merge/1
  Merge/1 -> Out1/1
  In Bus Element5/1 -> If Action Subsystem/1(hv)  "hv"
  In Bus Element4/1 -> If Action Subsystem1/1(hv)  "hv"

== system TVModel_Simulation_21/Subsystem/Subsystem1/Torque Distribution/MPC/USEFUL STUFFFF/Power flag ==
  Motor_Torque : Inport
  dynamics_data : Inport  Port=2
  Constant : Constant  Value=79000
  Constant1 : Constant  Value=0
  Constant2 : Constant  Value=-34000
  Efficiency limit : Subsystem
  Less Than : RelationalOperator  OutDataTypeStr=boolean  RndMeth=Simplest
  Less Than1 : RelationalOperator  OutDataTypeStr=boolean  RndMeth=Simplest
  Less Than2 : RelationalOperator  Operator=<=  OutDataTypeStr=boolean  RndMeth=Simplest
  Sum1 : Sum  Inputs=+
  Output : Outport
  wires:
  Motor_Torque/1 -> Efficiency limit/1(Motor_Torque)
  dynamics_data/1 -> Efficiency limit/2(dynamics_data)
  ? -> ?
  ? -> Sum1/1
  Efficiency limit/1(Limit) -> ?  "Limit"
  Constant/1 -> Less Than/2
  Constant1/1 -> Less Than1/2
  Constant2/1 -> Less Than2/2
  Sum1/1 -> Less Than/1, Less Than1/1, Less Than2/1  "Power"

== system TVModel_Simulation_21/Subsystem/Subsystem1/Torque Distribution/MPC/USEFUL STUFFFF/States Selector ==
  In1 : Inport
  Demux : Demux  Outputs=7
  Mux : Mux
  Selector : Selector  InputPortWidth=7  IndexOptions=Index vector (dialog)  Indices=[4:7]  OutputSizes=1
  Terminator : Terminator
  Terminator1 : Terminator
  Terminator2 : Terminator
  Control : Outport
  wires:
  Demux/3 -> Terminator2/1
  Demux/2 -> Terminator1/1
  Demux/1 -> Terminator/1
  Demux/5 -> Mux/2
  Demux/6 -> Mux/3
  Demux/7 -> Mux/4
  Demux/4 -> Mux/1
  In1/1 -> Selector/1, Demux/1
  Selector/1 -> Control/1

== system TVModel_Simulation_21/Subsystem/Subsystem1/Torque Distribution/MPC/USEFUL STUFFFF/Subsystem ==
  T : Inport
  In2 : Inport  Port=2
  In3 : Inport  Port=3
  Constant : Constant  Value=-35000
  Constant1 : Constant  Value=TV.LV.efficiency_LUT.Eta
  Constant2 : Constant  Value=TV.LV.efficiency_LUT.Omega
  Constant3 : Constant  Value=TV.LV.efficiency_LUT.Torque
  Constant4 : Constant  Value=TV.LV.GENERAL.BrakeThresh
  Constant5 : Constant  Value=80000
  Gain1 : Gain  Gain=TV.CAR.Tau
  Less Than1 : RelationalOperator  Operator=<  OutDataTypeStr=boolean  RndMeth=Simplest
  MATLAB Function : MATLAB Function  TreatAsAtomicUnit=on
  Switch1 : Switch  Criteria=u2 > Threshold
  Terminator1 : Terminator
  Terminator2 : Terminator
  Output : Outport
  wires:
  In3/1 -> Less Than1/2
  T/1 -> MATLAB Function/1(T)
  In2/1 -> Gain1/1
  Switch1/1 -> MATLAB Function/2(Plim)
  Less Than1/1 -> Switch1/2, MATLAB Function/7(brake_flag)
  Constant4/1 -> Less Than1/1
  MATLAB Function/1(Tnew) -> Output/1  "Tnew"
  MATLAB Function/2(k) -> Terminator1/1  "k"
  MATLAB Function/3(fx) -> Terminator2/1  "fx"
  Constant2/1 -> MATLAB Function/4(Omega)
  Constant3/1 -> MATLAB Function/5(Torque)
  Constant5/1 -> Switch1/3
  Constant/1 -> Switch1/1
  Constant1/1 -> MATLAB Function/3(Eta)
  Gain1/1 -> MATLAB Function/6(Omega_motors)

== system TVModel_Simulation_21/Subsystem/Subsystem1/Torque Distribution/MPC/USEFUL STUFFFF/Subsystem1 ==
  front_wheel_angles : Inport
  Steer Activation : Subsystem
  epsilon : Outport
  wires:
  front_wheel_angles/1 -> Steer Activation/1(front_wheel_angle)  "delta"
  Steer Activation/1(epsilon) -> epsilon/1

== system TVModel_Simulation_21/Subsystem/Subsystem1/Torque Distribution/MPC/USEFUL STUFFFF/Yrd 0 When Steering 0 ==
  yaw_rate_desired_LUT : Inport
  front_steer_angle : Inport  Port=2
  vx : Inport  Port=3
  Abs : Abs
  Constant5 : Constant  Value=0
  Linear Activation : MATLAB Function  TreatAsAtomicUnit=on
  Steer Limit : Subsystem
      mask Display: image('Mask_Icon\steering-wheel.png'); % Use "Edit Image" on toolstrip to change.
  yaw_rate_desired : Outport
  wires:
  Constant5/1 -> Linear Activation/3(in_2)
  yaw_rate_desired_LUT/1 -> Linear Activation/1(in_1)
  Linear Activation/1(out) -> yaw_rate_desired/1
  Steer Limit/1(steer_limit) -> Linear Activation/2(epsilon)
  front_steer_angle/1 -> Abs/1
  vx/1 -> Steer Limit/2(Inport)
  Abs/1 -> Steer Limit/1(front_wheel_angle)

== system TVModel_Simulation_21/Subsystem/Subsystem1/Torque Distribution/MPC/USEFUL STUFFFF/lbu_dot ==
  In Bus Element13 : Inport  PortName=brake_signal  Element=regen
  Motor_Torque : Inport  Port=2
  AND : Logic  IconShape=distinctive  AllPortsSameDT=off  OutDataTypeStr=boolean
  Constant6 : Constant  Value=-TV.LV.TORQUE.T_peak_motor
  Constant8 : Constant  Value=5
  Constant9 : Constant  Value=TV.LV.GENERAL.BrakeThresh
  Less Than3 : RelationalOperator  Operator=<  OutDataTypeStr=boolean  RndMeth=Simplest
  Less Than4 : RelationalOperator  Operator=<  OutDataTypeStr=boolean  RndMeth=Simplest
  Sum : Sum  Inputs=|+-
  Switch1 : Switch  Criteria=u2 > Threshold
  Unit Delay1 : UnitDelay  SampleTime=-1  HasFrameUpgradeWarning=on
  lbu_in : Outport
  wires:
  Less Than4/1 -> AND/2
  Less Than3/1 -> AND/1
  Unit Delay1/1 -> Less Than3/1
  Constant9/1 -> Less Than4/1, Less Than3/2
  In Bus Element13/1 -> Unit Delay1/1, Less Than4/2
  Constant8/1 -> Sum/2
  Sum/1 -> Switch1/3
  AND/1 -> Switch1/2
  Constant6/1 -> Switch1/1
  Switch1/1 -> lbu_in/1
  Motor_Torque/1 -> Sum/1

== system TVModel_Simulation_21/Subsystem/Subsystem1/Torque Distribution/MPC/Useful Calculations/Power Calculation Post ==
  In Bus Element34 : Inport  PortName=dynamics_data  Element=omega_wheels
  In Bus Element2 : Inport  PortName=dynamics_data  Element=omega_wheels
  Motor_Torque : Inport  Port=2  OutDataTypeStr=double  PortDimensions=4
  "     " : Gain  Gain=TV.LV.inv_efficiency
  "      " : Gain  Gain=1/TV.LV.inv_efficiency
  Divide : Product  Inputs=*/*
  Gain2 : Gain  Gain=TV.CAR.Tau
  Power to engines : Subsystem
  Saturation : Saturate  UpperLimit=19900*pi/30  LowerLimit=100*pi/30
  Sum of Elements : Sum  Inputs=+
  Switch3 : Switch  Criteria=u2 > Threshold
  Terminator : Terminator
  wires:
  Divide/1 -> Sum of Elements/1
  Saturation/1 -> Divide/1, Power to engines/1(omega_motor)
  Power to engines/1(Efficiency) -> "      "/1, "     "/1
  "      "/1 -> Switch3/3  "Braking"
  "     "/1 -> Switch3/1  "Driving"
  Motor_Torque/1 -> Power to engines/2(Torque), Divide/3
  In Bus Element34/1 -> Gain2/1
  Gain2/1 -> Saturation/1
  In Bus Element2/1 -> Switch3/2
  Switch3/1 -> Divide/2  "efficiency_new"
  Sum of Elements/1 -> Terminator/1  "p_el_post"

== system TVModel_Simulation_21/Subsystem/Subsystem1/Torque Distribution/MPC/Weights Generation/Efficiency limit ==
  motor_torque : Inport  OutDataTypeStr=double  PortDimensions=4
  In Bus Element34 : Inport  Port=2  PortName=dynamics_data  Element=omega_wheels
  In Bus Element2 : Inport  Port=2  PortName=dynamics_data  Element=omega_wheels
  In Bus Element1 : Inport  Port=2  PortName=dynamics_data  Element=omega_wheels
  "     " : Gain  Gain=TV.LV.inv_efficiency
  "      " : Gain  Gain=1/TV.LV.inv_efficiency
  Gain1 : Gain  Gain=TV.CAR.Tau
  Gain2 : Gain  Gain=TV.CAR.Tau
  Power to engines : Subsystem
  Product : Product
  Saturation : Saturate  UpperLimit=19900*pi/30  LowerLimit=100*pi/30
  Switch3 : Switch  Criteria=u2 > Threshold
  efficiency_limit : Outport
  wires:
  Gain1/1 -> Product/1
  Product/1 -> efficiency_limit/1
  In Bus Element1/1 -> Gain1/1
  Power to engines/1(Efficiency) -> "      "/1, "     "/1
  "      "/1 -> Switch3/3  "Braking"
  "     "/1 -> Switch3/1  "Driving"
  motor_torque/1 -> Power to engines/2(Torque)
  In Bus Element34/1 -> Gain2/1
  Gain2/1 -> Saturation/1
  In Bus Element2/1 -> Switch3/2
  Saturation/1 -> Power to engines/1(omega_motor)
  Switch3/1 -> Product/2

== system TVModel_Simulation_21/Subsystem/Subsystem1/Slip Control/Traction Control/ABS/Load Transfer Calculation1/Fz FL ==
  In Bus Element : Inport  PortName=dynamics_data  Element=ay
  In Bus Element1 : Inport  PortName=dynamics_data  Element=vx
  In Bus Element2 : Inport  PortName=dynamics_data  Element=ax
  Drag moment : Gain  Gain=0.5*TV.CAR.rho*TV.CAR.CdA*TV.CAR.hcop/TV.CAR.wb*0.5
  Lateral Load Transfer : Gain  Gain=TV.CAR.m/TV.CAR.tf*TV.CAR.hcog*0.5
  Lift Force : Gain  Gain=0.5*TV.CAR.rho*TV.CAR.ClA*(1-TV.CAR.xcop/TV.CAR.wb)*0.5
  Longitudinal Load Transfer : Gain  Gain=TV.CAR.m/TV.CAR.wb*TV.CAR.hcog*0.5
  Square1 : Math  Operator=square  SaturateOnIntegerOverflow=on
  Square2 : Math  Operator=square  SaturateOnIntegerOverflow=on
  Static Load Front : Constant  Value=TV.CAR.Fzf
  Subtract : Sum  Inputs=+++-+
  Unary Minus : UnaryMinus
  Unary Minus1 : UnaryMinus
  TV_Info : Outport
  wires:
  Lift Force/1 -> Subtract/3
  In Bus Element1/1 -> Square1/1, Square2/1
  Square2/1 -> Drag moment/1
  In Bus Element2/1 -> Unary Minus1/1
  Longitudinal Load Transfer/1 -> Subtract/5
  Lateral Load Transfer/1 -> Subtract/2
  Square1/1 -> Lift Force/1
  Static Load Front/1 -> Subtract/1
  Drag moment/1 -> Subtract/4
  Subtract/1 -> TV_Info/1
  In Bus Element/1 -> Unary Minus/1
  Unary Minus/1 -> Lateral Load Transfer/1
  Unary Minus1/1 -> Longitudinal Load Transfer/1

== system TVModel_Simulation_21/Subsystem/Subsystem1/Slip Control/Traction Control/ABS/Load Transfer Calculation1/Fz FR ==
  In Bus Element : Inport  PortName=dynamics_data  Element=ay
  In Bus Element1 : Inport  PortName=dynamics_data  Element=vx
  In Bus Element2 : Inport  PortName=dynamics_data  Element=ax
  Drag moment : Gain  Gain=0.5*TV.CAR.rho*TV.CAR.CdA*TV.CAR.hcop/TV.CAR.wb*0.5
  Lateral Load Transfer : Gain  Gain=TV.CAR.m/TV.CAR.tf*TV.CAR.hcog*0.5
  Lift Force : Gain  Gain=0.5*TV.CAR.rho*TV.CAR.ClA*(1 - TV.CAR.xcop/TV.CAR.wb)*0.5
  Longitudinal Load Transfer : Gain  Gain=TV.CAR.m/TV.CAR.wb*TV.CAR.hcog*0.5
  Square1 : Math  Operator=square  SaturateOnIntegerOverflow=on
  Square2 : Math  Operator=square  SaturateOnIntegerOverflow=on
  Static Load Front : Constant  Value=TV.CAR.Fzf
  Subtract : Sum  Inputs=+-+-+
  Unary Minus : UnaryMinus
  Unary Minus1 : UnaryMinus
  TV_Info : Outport
  wires:
  Square2/1 -> Drag moment/1
  Lift Force/1 -> Subtract/3
  In Bus Element2/1 -> Unary Minus1/1
  Longitudinal Load Transfer/1 -> Subtract/5
  Lateral Load Transfer/1 -> Subtract/2
  Square1/1 -> Lift Force/1
  Static Load Front/1 -> Subtract/1
  In Bus Element1/1 -> Square2/1, Square1/1
  In Bus Element/1 -> Unary Minus/1
  Drag moment/1 -> Subtract/4
  Subtract/1 -> TV_Info/1
  Unary Minus/1 -> Lateral Load Transfer/1
  Unary Minus1/1 -> Longitudinal Load Transfer/1

== system TVModel_Simulation_21/Subsystem/Subsystem1/Slip Control/Traction Control/ABS/Load Transfer Calculation1/Fz RL ==
  In Bus Element : Inport  PortName=dynamics_data  Element=ay
  In Bus Element1 : Inport  PortName=dynamics_data  Element=vx
  In Bus Element2 : Inport  PortName=dynamics_data  Element=ax
  Drag moment : Gain  Gain=0.5*TV.CAR.rho*TV.CAR.CdA*TV.CAR.hcop/TV.CAR.wb*0.5
  Lateral Load Transfer : Gain  Gain=TV.CAR.m/TV.CAR.tr*TV.CAR.hcog*0.5
  Lift Force : Gain  Gain=0.5*TV.CAR.rho*TV.CAR.ClA*(TV.CAR.xcop/TV.CAR.wb)*0.5
  Longitudinal Load Transfer : Gain  Gain=TV.CAR.m/TV.CAR.wb*TV.CAR.hcog*0.5
  Square1 : Math  Operator=square  SaturateOnIntegerOverflow=on
  Square2 : Math  Operator=square  SaturateOnIntegerOverflow=on
  Static Load Front : Constant  Value=TV.CAR.Fzr
  Subtract : Sum  Inputs=++++-
  Unary Minus : UnaryMinus
  Unary Minus1 : UnaryMinus
  TV_Info : Outport
  wires:
  In Bus Element1/1 -> Square1/1, Square2/1
  Square2/1 -> Drag moment/1
  Lift Force/1 -> Subtract/3
  In Bus Element2/1 -> Unary Minus1/1
  Longitudinal Load Transfer/1 -> Subtract/5
  Lateral Load Transfer/1 -> Subtract/2
  Square1/1 -> Lift Force/1
  Static Load Front/1 -> Subtract/1
  In Bus Element/1 -> Unary Minus/1
  Drag moment/1 -> Subtract/4
  Subtract/1 -> TV_Info/1
  Unary Minus/1 -> Lateral Load Transfer/1
  Unary Minus1/1 -> Longitudinal Load Transfer/1

== system TVModel_Simulation_21/Subsystem/Subsystem1/Slip Control/Traction Control/ABS/Load Transfer Calculation1/Fz RR ==
  In Bus Element : Inport  PortName=dynamics_data  Element=ay
  In Bus Element1 : Inport  PortName=dynamics_data  Element=vx
  In Bus Element2 : Inport  PortName=dynamics_data  Element=ax
  Drag moment : Gain  Gain=0.5*TV.CAR.rho*TV.CAR.CdA*TV.CAR.hcop/TV.CAR.wb*0.5
  Lateral Load Transfer : Gain  Gain=TV.CAR.m/TV.CAR.tr*TV.CAR.hcog*0.5
  Lift Force : Gain  Gain=0.5*TV.CAR.rho*TV.CAR.ClA*(TV.CAR.xcop/TV.CAR.wb)*0.5
  Longitudinal Load Transfer : Gain  Gain=TV.CAR.m/TV.CAR.wb*TV.CAR.hcog*0.5
  Square1 : Math  Operator=square  SaturateOnIntegerOverflow=on
  Square2 : Math  Operator=square  SaturateOnIntegerOverflow=on
  Static Load Front : Constant  Value=TV.CAR.Fzr
  Subtract : Sum  Inputs=+-++-
  Unary Minus : UnaryMinus
  Unary Minus1 : UnaryMinus
  TV_Info : Outport
  wires:
  Square2/1 -> Drag moment/1
  Lift Force/1 -> Subtract/3
  In Bus Element2/1 -> Unary Minus1/1
  Longitudinal Load Transfer/1 -> Subtract/5
  Lateral Load Transfer/1 -> Subtract/2
  Square1/1 -> Lift Force/1
  Static Load Front/1 -> Subtract/1
  In Bus Element1/1 -> Square2/1, Square1/1
  In Bus Element/1 -> Unary Minus/1
  Drag moment/1 -> Subtract/4
  Subtract/1 -> TV_Info/1
  Unary Minus/1 -> Lateral Load Transfer/1
  Unary Minus1/1 -> Longitudinal Load Transfer/1

== system TVModel_Simulation_21/Subsystem/Subsystem1/Slip Control/Traction Control/Slip Control/epsTarget computation/kappaTarget selection ==
  alphaWheel : Inport
  Constant : Constant  Value=2
  If Action Subsystem : Subsystem  TreatAsAtomicUnit=on
  If Action Subsystem1 : Subsystem  TreatAsAtomicUnit=on
  If Action Subsystem2 : Subsystem  TreatAsAtomicUnit=on
  If Action Subsystem3 : Subsystem  TreatAsAtomicUnit=on
  Merge : Merge  Inputs=4
  Switch Case : SwitchCase  CaseConditions={1,2,3,4}  ShowDefaultCase=off
  kappaTarget : Outport
  wires:
  Merge/1 -> kappaTarget/1
  If Action Subsystem3/1(Out1) -> Merge/4
  If Action Subsystem2/1(Out1) -> Merge/3
  If Action Subsystem1/1(Out1) -> Merge/2
  If Action Subsystem/1(Out1) -> Merge/1
  [sr98] -> If Action Subsystem3/Action
  [sr95] -> If Action Subsystem2/Action
  [sr93] -> If Action Subsystem1/Action
  [sr90] -> If Action Subsystem/Action
  alphaWheel/1 -> If Action Subsystem/1(alphaWheel), If Action Subsystem1/1(alphaWheel), If Action Subsystem2/1(alphaWheel), If Action Subsystem3/1(alphaWheel)
  Constant/1 -> Switch Case/1
  Switch Case/4 -> [sr98]
  Switch Case/3 -> [sr95]
  Switch Case/2 -> [sr93]
  Switch Case/1 -> [sr90]

== system TVModel_Simulation_21/Subsystem/Subsystem1/Slip Control/Traction Control/TC/Load Transfer Calculation1/Fz FL ==
  In Bus Element : Inport  PortName=dynamics_data  Element=ay
  In Bus Element1 : Inport  PortName=dynamics_data  Element=vx
  In Bus Element2 : Inport  PortName=dynamics_data  Element=ax
  Drag moment : Gain  Gain=0.5*TV.CAR.rho*TV.CAR.CdA*TV.CAR.hcop/TV.CAR.wb*0.5
  Lateral Load Transfer : Gain  Gain=TV.CAR.m/TV.CAR.tf*TV.CAR.hcog*0.5
  Lift Force : Gain  Gain=0.5*TV.CAR.rho*TV.CAR.ClA*(1-TV.CAR.xcop/TV.CAR.wb)*0.5
  Longitudinal Load Transfer : Gain  Gain=TV.CAR.m/TV.CAR.wb*TV.CAR.hcog*0.5
  Square1 : Math  Operator=square  SaturateOnIntegerOverflow=on
  Square2 : Math  Operator=square  SaturateOnIntegerOverflow=on
  Static Load Front : Constant  Value=TV.CAR.Fzf
  Subtract : Sum  Inputs=+++-+
  Unary Minus : UnaryMinus
  Unary Minus1 : UnaryMinus
  TV_Info : Outport
  wires:
  Unary Minus1/1 -> Longitudinal Load Transfer/1
  Unary Minus/1 -> Lateral Load Transfer/1
  In Bus Element/1 -> Unary Minus/1
  Subtract/1 -> TV_Info/1
  Drag moment/1 -> Subtract/4
  Static Load Front/1 -> Subtract/1
  Square1/1 -> Lift Force/1
  Lateral Load Transfer/1 -> Subtract/2
  Longitudinal Load Transfer/1 -> Subtract/5
  In Bus Element2/1 -> Unary Minus1/1
  Square2/1 -> Drag moment/1
  In Bus Element1/1 -> Square2/1, Square1/1
  Lift Force/1 -> Subtract/3

== system TVModel_Simulation_21/Subsystem/Subsystem1/Slip Control/Traction Control/TC/Load Transfer Calculation1/Fz FR ==
  In Bus Element : Inport  PortName=dynamics_data  Element=ay
  In Bus Element1 : Inport  PortName=dynamics_data  Element=vx
  In Bus Element2 : Inport  PortName=dynamics_data  Element=ax
  Drag moment : Gain  Gain=0.5*TV.CAR.rho*TV.CAR.CdA*TV.CAR.hcop/TV.CAR.wb*0.5
  Lateral Load Transfer : Gain  Gain=TV.CAR.m/TV.CAR.tf*TV.CAR.hcog*0.5
  Lift Force : Gain  Gain=0.5*TV.CAR.rho*TV.CAR.ClA*(1 - TV.CAR.xcop/TV.CAR.wb)*0.5
  Longitudinal Load Transfer : Gain  Gain=TV.CAR.m/TV.CAR.wb*TV.CAR.hcog*0.5
  Square1 : Math  Operator=square  SaturateOnIntegerOverflow=on
  Square2 : Math  Operator=square  SaturateOnIntegerOverflow=on
  Static Load Front : Constant  Value=TV.CAR.Fzf
  Subtract : Sum  Inputs=+-+-+
  Unary Minus : UnaryMinus
  Unary Minus1 : UnaryMinus
  TV_Info : Outport
  wires:
  Unary Minus1/1 -> Longitudinal Load Transfer/1
  Unary Minus/1 -> Lateral Load Transfer/1
  Subtract/1 -> TV_Info/1
  Drag moment/1 -> Subtract/4
  In Bus Element/1 -> Unary Minus/1
  In Bus Element1/1 -> Square1/1, Square2/1
  Static Load Front/1 -> Subtract/1
  Square1/1 -> Lift Force/1
  Lateral Load Transfer/1 -> Subtract/2
  Longitudinal Load Transfer/1 -> Subtract/5
  In Bus Element2/1 -> Unary Minus1/1
  Lift Force/1 -> Subtract/3
  Square2/1 -> Drag moment/1

== system TVModel_Simulation_21/Subsystem/Subsystem1/Slip Control/Traction Control/TC/Load Transfer Calculation1/Fz RL ==
  In Bus Element : Inport  PortName=dynamics_data  Element=ay
  In Bus Element1 : Inport  PortName=dynamics_data  Element=vx
  In Bus Element2 : Inport  PortName=dynamics_data  Element=ax
  Drag moment : Gain  Gain=0.5*TV.CAR.rho*TV.CAR.CdA*TV.CAR.hcop/TV.CAR.wb*0.5
  Lateral Load Transfer : Gain  Gain=TV.CAR.m/TV.CAR.tr*TV.CAR.hcog*0.5
  Lift Force : Gain  Gain=0.5*TV.CAR.rho*TV.CAR.ClA*(TV.CAR.xcop/TV.CAR.wb)*0.5
  Longitudinal Load Transfer : Gain  Gain=TV.CAR.m/TV.CAR.wb*TV.CAR.hcog*0.5
  Square1 : Math  Operator=square  SaturateOnIntegerOverflow=on
  Square2 : Math  Operator=square  SaturateOnIntegerOverflow=on
  Static Load Front : Constant  Value=TV.CAR.Fzr
  Subtract : Sum  Inputs=++++-
  Unary Minus : UnaryMinus
  Unary Minus1 : UnaryMinus
  TV_Info : Outport
  wires:
  Unary Minus1/1 -> Longitudinal Load Transfer/1
  Unary Minus/1 -> Lateral Load Transfer/1
  Subtract/1 -> TV_Info/1
  Drag moment/1 -> Subtract/4
  In Bus Element/1 -> Unary Minus/1
  Static Load Front/1 -> Subtract/1
  Square1/1 -> Lift Force/1
  Lateral Load Transfer/1 -> Subtract/2
  Longitudinal Load Transfer/1 -> Subtract/5
  In Bus Element2/1 -> Unary Minus1/1
  Lift Force/1 -> Subtract/3
  Square2/1 -> Drag moment/1
  In Bus Element1/1 -> Square2/1, Square1/1

== system TVModel_Simulation_21/Subsystem/Subsystem1/Slip Control/Traction Control/TC/Load Transfer Calculation1/Fz RR ==
  In Bus Element : Inport  PortName=dynamics_data  Element=ay
  In Bus Element1 : Inport  PortName=dynamics_data  Element=vx
  In Bus Element2 : Inport  PortName=dynamics_data  Element=ax
  Drag moment : Gain  Gain=0.5*TV.CAR.rho*TV.CAR.CdA*TV.CAR.hcop/TV.CAR.wb*0.5
  Lateral Load Transfer : Gain  Gain=TV.CAR.m/TV.CAR.tr*TV.CAR.hcog*0.5
  Lift Force : Gain  Gain=0.5*TV.CAR.rho*TV.CAR.ClA*(TV.CAR.xcop/TV.CAR.wb)*0.5
  Longitudinal Load Transfer : Gain  Gain=TV.CAR.m/TV.CAR.wb*TV.CAR.hcog*0.5
  Square1 : Math  Operator=square  SaturateOnIntegerOverflow=on
  Square2 : Math  Operator=square  SaturateOnIntegerOverflow=on
  Static Load Front : Constant  Value=TV.CAR.Fzr
  Subtract : Sum  Inputs=+-++-
  Unary Minus : UnaryMinus
  Unary Minus1 : UnaryMinus
  TV_Info : Outport
  wires:
  Unary Minus1/1 -> Longitudinal Load Transfer/1
  Unary Minus/1 -> Lateral Load Transfer/1
  Subtract/1 -> TV_Info/1
  Drag moment/1 -> Subtract/4
  In Bus Element/1 -> Unary Minus/1
  In Bus Element1/1 -> Square1/1, Square2/1
  Static Load Front/1 -> Subtract/1
  Square1/1 -> Lift Force/1
  Lateral Load Transfer/1 -> Subtract/2
  Longitudinal Load Transfer/1 -> Subtract/5
  In Bus Element2/1 -> Unary Minus1/1
  Lift Force/1 -> Subtract/3
  Square2/1 -> Drag moment/1

== system TVModel_Simulation_21/Subsystem/Subsystem1/Torque Distribution/MPC/ PRE LUDO/Faul Detection/MPC ==
  In1 : Inport
  Action Port : ActionPort
  Out1 : Outport
  wires:
  In1/1 -> Out1/1

== system TVModel_Simulation_21/Subsystem/Subsystem1/Torque Distribution/MPC/ PRE LUDO/Faul Detection/Simple torque ==
  Action Port : ActionPort
